simulink model "identifikalt_modell2"  (R2024b)
settings: Solver=VariableStepAuto  StartTime=0.0  StopTime=20  RelTol=1e-3
values from neighbouring files (symbols this model uses):
  Ft1 = Phit1-Gtilde1*Ct1*Phit1    [ident_test.m]
  Ft2 = Phit2-Gtilde2*Ct2*Phit2    [ident_test.m]
  Gtilde1 = acker(Phit1',Phit1'*Ct1',[zcinf1 zcinf1 zcinf1 zcinf1]')'    [ident_test.m]
  Gtilde2 = acker(Phit2',Phit2'*Ct2',[zcinf2 zcinf2 zcinf2 zcinf2]')'    [ident_test.m]
  Ht1 = Gammat1-Gtilde1*Ct1*Gammat1    [ident_test.m]
  Ht2 = Gammat2-Gtilde2*Ct2*Gammat2    [ident_test.m]
  K1 = acker(Phi1,Gamma1,[z1 z1c zoinf1])    [ident_test.m]
  K2 = acker(Phi2,Gamma2,[z2 z2c zoinf2])    [ident_test.m]
  linear_sys_ss1 = ss(nlhw1.LinearModel)    [ident_test.m]
  linear_sys_ss2 = ss(nlhw2.LinearModel)    [ident_test.m]
  Nu1 = N1(4)    [ident_test.m]
  Nu2 = N2(4)    [ident_test.m]
  Nx1 = N1(1:3)    [ident_test.m]
  Nx2 = N2(1:3)    [ident_test.m]
libraries: simulink x1
settings Model: Creator=Asus  LastModifiedBy=Asus

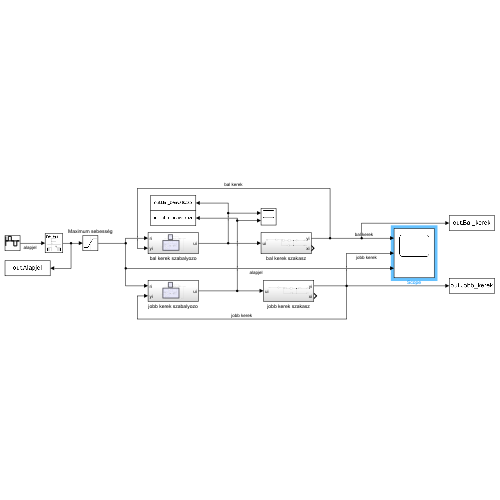
[thumbnail: Simulink's stored preview of the top-level diagram]
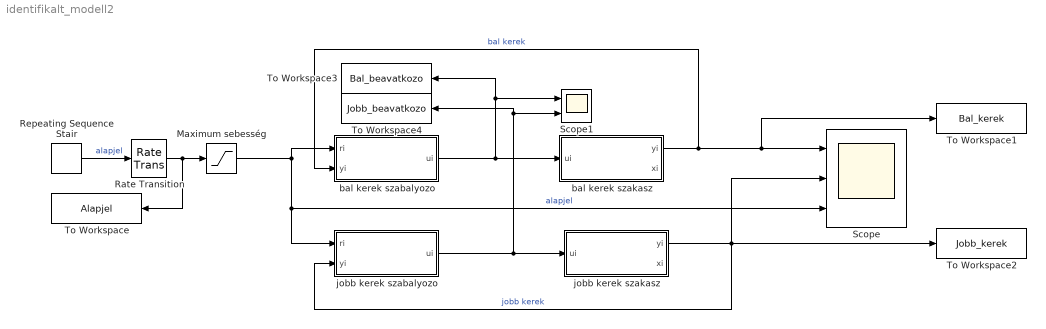
== system identifikalt_modell2 ==
  Maximum sebesség : Saturate  UpperLimit=0.6  LowerLimit=-0.6
  Rate Transition : RateTransition  Deterministic=off  OutPortSampleTime=0.02
  Repeating Sequence Stair : simulink/Sources/Repeating Sequence Stair  OutValues=[0 0.15 0 -0.15 0].'  tsamp=5  OutMin=[]  OutMax=[]  OutDataTypeStr=double  OutputDataTypeScalingMode=double  OutDataType=fixdt(0,8)  ConRadixGroup=Best Precision: Vector-wise  OutScaling=2^-12
  Scope : Scope  NumInputPorts=3
  Scope1 : Scope  NumInputPorts=2
  To Workspace : ToWorkspace  VariableName=Alapjel  SaveFormat=Timeseries  SampleTime=-1
  To Workspace1 : ToWorkspace  VariableName=Bal_kerek  SaveFormat=Timeseries  SampleTime=-1
  To Workspace2 : ToWorkspace  VariableName=Jobb_kerek  SaveFormat=Timeseries  SampleTime=-1
  To Workspace3 : ToWorkspace  VariableName=Bal_beavatkozo  SaveFormat=Timeseries  SampleTime=-1
  To Workspace4 : ToWorkspace  VariableName=Jobb_beavatkozo  SaveFormat=Timeseries  SampleTime=-1
  bal kerek szabalyozo : Subsystem
  bal kerek szakasz : Subsystem
  jobb kerek szabalyozo : Subsystem
  jobb kerek szakasz : Subsystem
  wires:
  bal kerek szakasz/1(yi) -> bal kerek szabalyozo/2(yi), Scope/1, To Workspace1/1  "bal kerek"
  jobb kerek szakasz/1(yi) -> jobb kerek szabalyozo/2(yi), Scope/2, To Workspace2/1  "jobb kerek"
  Repeating Sequence Stair/1 -> Rate Transition/1  "alapjel"
  Maximum sebesség/1 -> bal kerek szabalyozo/1(ri), jobb kerek szabalyozo/1(ri), Scope/3  "alapjel"
  jobb kerek szabalyozo/1(ui) -> To Workspace4/1, Scope1/2, jobb kerek szakasz/1(ui)
  Rate Transition/1 -> Maximum sebesség/1, To Workspace/1
  bal kerek szabalyozo/1(ui) -> bal kerek szakasz/1(ui), To Workspace3/1, Scope1/1

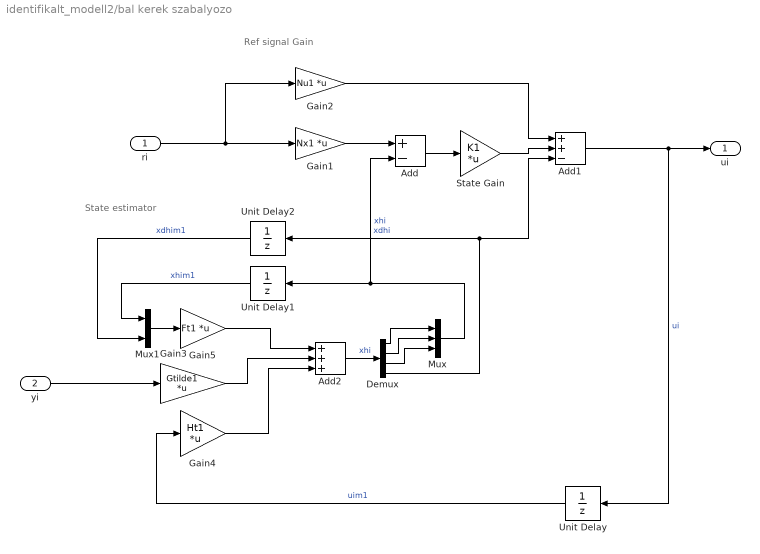
== system identifikalt_modell2/bal kerek szabalyozo ==
  note: Ref signal Gain
  note: State estimator
  ri : Inport
  yi : Inport  Port=2
  Add : Sum  Inputs=+-
  Add1 : Sum  Inputs=++-
  Add2 : Sum  Inputs=+++
  Demux : Demux
  Gain1 : Gain  Gain=Nx1  Multiplication=Matrix(K*u)
  Gain2 : Gain  Gain=Nu1  Multiplication=Matrix(K*u)
  Gain3 : Gain  Gain=Gtilde1  Multiplication=Matrix(K*u)
  Gain4 : Gain  Gain=Ht1  Multiplication=Matrix(K*u)
  Gain5 : Gain  Gain=Ft1  Multiplication=Matrix(K*u)
  Mux : Mux  Inputs=3
  Mux1 : Mux  Inputs=2
  State Gain : Gain  Gain=K1  Multiplication=Matrix(K*u)
  Unit Delay : UnitDelay  SampleTime=-1  HasFrameUpgradeWarning=on
  Unit Delay1 : UnitDelay  SampleTime=-1  HasFrameUpgradeWarning=on
  Unit Delay2 : UnitDelay  SampleTime=-1  HasFrameUpgradeWarning=on
  ui : Outport
  wires:
  Add/1 -> State Gain/1
  Mux/1 -> Unit Delay1/1, Add/2  "xhi"
  ri/1 -> Gain1/1, Gain2/1
  Add1/1 -> Unit Delay/1, ui/1  "ui"
  State Gain/1 -> Add1/2
  Gain1/1 -> Add/1
  Gain2/1 -> Add1/1
  yi/1 -> Gain3/1
  Gain4/1 -> Add2/3
  Gain3/1 -> Add2/2
  Unit Delay/1 -> Gain4/1  "uim1"
  Gain5/1 -> Add2/1
  Unit Delay1/1 -> Mux1/1  "xhim1"
  Add2/1 -> Demux/1  "xhi"
  Demux/1 -> Mux/1
  Demux/2 -> Mux/2
  Demux/3 -> Mux/3
  Demux/4 -> Add1/3, Unit Delay2/1  "xdhi"
  Mux1/1 -> Gain5/1
  Unit Delay2/1 -> Mux1/2  "xdhim1"

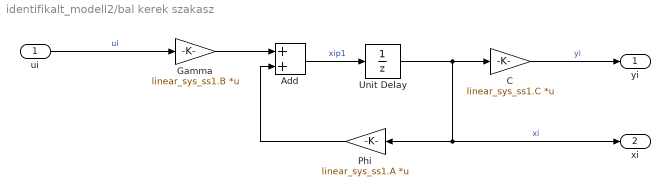
== system identifikalt_modell2/bal kerek szakasz ==
  ui : Inport
  Add : Sum
  C : Gain  Gain=linear_sys_ss1.C  Multiplication=Matrix(K*u)
  Gamma : Gain  Gain=linear_sys_ss1.B  Multiplication=Matrix(K*u)
  Phi : Gain  Gain=linear_sys_ss1.A  Multiplication=Matrix(K*u)
  Unit Delay : UnitDelay  SampleTime=0.02  HasFrameUpgradeWarning=on
  yi : Outport
  xi : Outport  Port=2
  wires:
  ui/1 -> Gamma/1  "ui"
  Gamma/1 -> Add/1
  C/1 -> yi/1  "yi"
  Unit Delay/1 -> xi/1, Phi/1, C/1  "xi"
  Add/1 -> Unit Delay/1  "xip1"
  Phi/1 -> Add/2

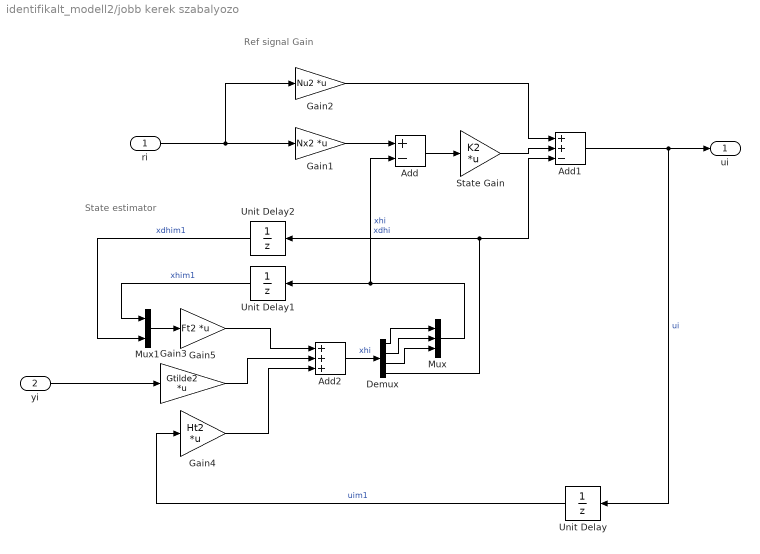
== system identifikalt_modell2/jobb kerek szabalyozo ==
  note: Ref signal Gain
  note: State estimator
  ri : Inport
  yi : Inport  Port=2
  Add : Sum  Inputs=+-
  Add1 : Sum  Inputs=++-
  Add2 : Sum  Inputs=+++
  Demux : Demux
  Gain1 : Gain  Gain=Nx2  Multiplication=Matrix(K*u)
  Gain2 : Gain  Gain=Nu2  Multiplication=Matrix(K*u)
  Gain3 : Gain  Gain=Gtilde2  Multiplication=Matrix(K*u)
  Gain4 : Gain  Gain=Ht2  Multiplication=Matrix(K*u)
  Gain5 : Gain  Gain=Ft2  Multiplication=Matrix(K*u)
  Mux : Mux  Inputs=3
  Mux1 : Mux  Inputs=2
  State Gain : Gain  Gain=K2  Multiplication=Matrix(K*u)
  Unit Delay : UnitDelay  SampleTime=-1  HasFrameUpgradeWarning=on
  Unit Delay1 : UnitDelay  SampleTime=-1  HasFrameUpgradeWarning=on
  Unit Delay2 : UnitDelay  SampleTime=-1  HasFrameUpgradeWarning=on
  ui : Outport
  wires:
  Add/1 -> State Gain/1
  Mux/1 -> Unit Delay1/1, Add/2  "xhi"
  ri/1 -> Gain1/1, Gain2/1
  Add1/1 -> Unit Delay/1, ui/1  "ui"
  State Gain/1 -> Add1/2
  Gain1/1 -> Add/1
  Gain2/1 -> Add1/1
  yi/1 -> Gain3/1
  Gain4/1 -> Add2/3
  Gain3/1 -> Add2/2
  Unit Delay/1 -> Gain4/1  "uim1"
  Gain5/1 -> Add2/1
  Unit Delay1/1 -> Mux1/1  "xhim1"
  Add2/1 -> Demux/1  "xhi"
  Demux/1 -> Mux/1
  Demux/2 -> Mux/2
  Demux/3 -> Mux/3
  Demux/4 -> Add1/3, Unit Delay2/1  "xdhi"
  Mux1/1 -> Gain5/1
  Unit Delay2/1 -> Mux1/2  "xdhim1"

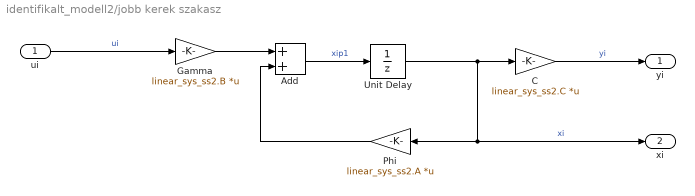
== system identifikalt_modell2/jobb kerek szakasz ==
  ui : Inport
  Add : Sum
  C : Gain  Gain=linear_sys_ss2.C  Multiplication=Matrix(K*u)
  Gamma : Gain  Gain=linear_sys_ss2.B  Multiplication=Matrix(K*u)
  Phi : Gain  Gain=linear_sys_ss2.A  Multiplication=Matrix(K*u)
  Unit Delay : UnitDelay  SampleTime=0.02  HasFrameUpgradeWarning=on
  yi : Outport
  xi : Outport  Port=2
  wires:
  ui/1 -> Gamma/1  "ui"
  Gamma/1 -> Add/1
  C/1 -> yi/1  "yi"
  Add/1 -> Unit Delay/1  "xip1"
  Phi/1 -> Add/2
  Unit Delay/1 -> xi/1, Phi/1, C/1  "xi"
